simulink model "FLIGHT_Hexacopter_V2"  (R2025a)
settings: Solver=FixedStepDiscrete  StartTime=0.0  StopTime=inf  FixedStep=SampleTime_SAS  RelTol=1e-3  EnableMultiTasking=on
InitFcn:
  | Init_FLIGHT_Hexacopter
values from neighbouring files (symbols this model uses):
  d2r = pi/180    (= 0.0174532925199)    [Init_FLIGHT_Hexacopter.m]
  Kdrr = 0.004    [Init_FLIGHT_Hexacopter_fromNCMS.m]
  Kirr = 0.0    (= 0)    [Init_FLIGHT_Hexacopter_fromNCMS.m]
  Kpp = 3.3894    [Init_FLIGHT_Hexacopter_fromNCMS.m]
  Kpr = 3.3894    [Init_FLIGHT_Hexacopter_fromNCMS.m]
  Kprr = 0.1    [Init_FLIGHT_Hexacopter_fromNCMS.m]
  MAX_CONTROL_ANGLE_PITCH = 30*pi/180    (= 0.523598775598)    [Init_FLIGHT_Hexacopter.m]    (also in Init_FLIGHT_Hexacopter_fromNCMS.m = 0.349065850399)
  MAX_CONTROL_ANGLE_RATE_PITCH = 360*pi/180    (= 6.28318530718)    [Init_FLIGHT_Hexacopter.m]    (also in Init_FLIGHT_Hexacopter_fromNCMS.m)
  MAX_CONTROL_ANGLE_RATE_ROLL = 360*pi/180    (= 6.28318530718)    [Init_FLIGHT_Hexacopter.m]    (also in Init_FLIGHT_Hexacopter_fromNCMS.m)
  MAX_CONTROL_ANGLE_RATE_Y = 120*pi/180    (= 2.09439510239)    [Init_FLIGHT_Hexacopter.m]    (also in Init_FLIGHT_Hexacopter_fromNCMS.m)
  MAX_CONTROL_ANGLE_ROLL = 30*pi/180    (= 0.523598775598)    [Init_FLIGHT_Hexacopter.m]    (also in Init_FLIGHT_Hexacopter_fromNCMS.m = 0.349065850399)
  Nrr = 50    [Init_FLIGHT_Hexacopter_fromNCMS.m]
  PITCH_AUTHORITY = 1    [Init_FLIGHT_Hexacopter.m]
  ROLL_AUTHORITY = 1    [Init_FLIGHT_Hexacopter.m]
  SampleTime = 1/250    (= 0.004)    [Init_FLIGHT_Hexacopter.m]    (also in Init_FLIGHT_Hexacopter_fromNCMS.m = 0.01)
  SampleTime_SAS = 1/1000    (= 0.001)    [Init_FLIGHT_Hexacopter.m]
  YAW_AUTHORITY = 1    [Init_FLIGHT_Hexacopter.m]
undefined symbols (not defined in the file or in its folder): arguments, DiscIntNeverNeededParam, e_dot, event_sequence, fx, g1x, hx, id, integral_e, log_levels, MPC_Z_D, MPC_Z_I, MPC_Z_P, noutputs, omega, omega_dot, output, phi_cmd, phi_cmd_ddot, phi_cmd_dot, r, s, tau_roll, timestamp, w
libraries: px4Utilslib x65, simulink x21, px4uORBlib x12, slpidlib x9, cstblocks x5, simulink_extras x2, sharedtransform x1, px4Sensorslib x1, matrix_library x1, px4Peripheralslib x1
(part 3 of 3)

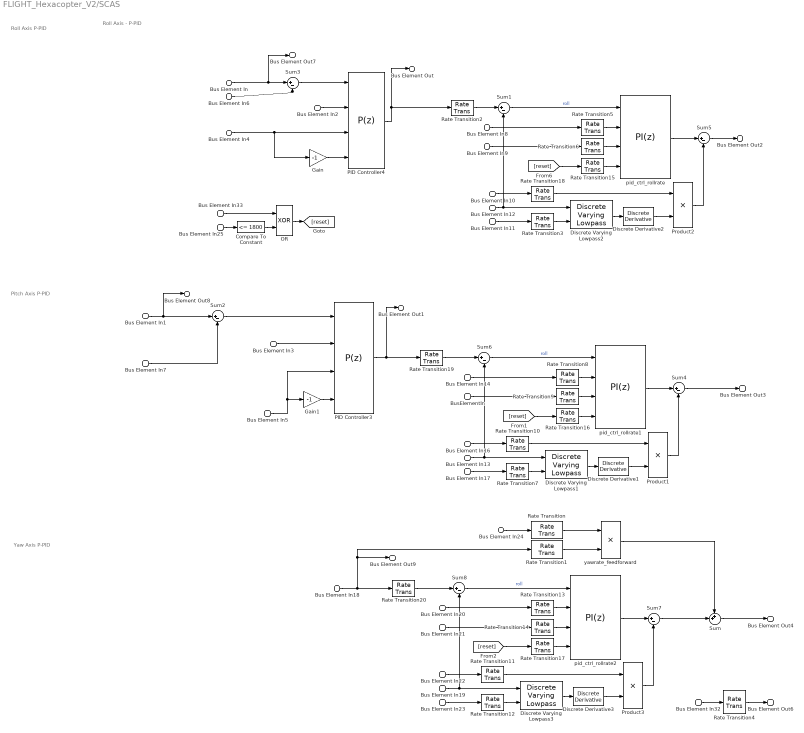
== system FLIGHT_Hexacopter_V2/SCAS ==
  note: Roll Axis P-PID
  note: Roll Axis - P-PID
  note: Pitch Axis P-PID
  note: Yaw Axis P-PID
  Bus Element In : Inport  PortName=OFP  Element=des_roll
  Bus Element In1 : Inport  PortName=OFP  Element=des_pitch
  Bus Element In18 : Inport  PortName=OFP  Element=des_yr
  Bus Element In32 : Inport  PortName=OFP  Element=des_thr
  Bus Element In2 : Inport  Port=2  PortName=PARAMS  Element=MC_ROLL_P
  Bus Element In3 : Inport  Port=2  PortName=PARAMS  Element=MC_PITCH_P
  Bus Element In4 : Inport  Port=2  PortName=PARAMS  Element=MC_ROLLRATE_MAX
  Bus Element In5 : Inport  Port=2  PortName=PARAMS  Element=MC_PITCHRATE_MAX
  Bus Element In8 : Inport  Port=2  PortName=PARAMS  Element=MC_ROLLRATE_P
  Bus Element In9 : Inport  Port=2  PortName=PARAMS  Element=MC_ROLLRATE_I
  Bus Element In10 : Inport  Port=2  PortName=PARAMS  Element=MC_ROLLRATE_D
  Bus Element In11 : Inport  Port=2  PortName=PARAMS  Element=IMU_DGYRO_CUTOFF
  Bus Element In17 : Inport  Port=2  PortName=PARAMS  Element=IMU_DGYRO_CUTOFF
  Bus Element In23 : Inport  Port=2  PortName=PARAMS  Element=IMU_DGYRO_CUTOFF
  Bus Element In14 : Inport  Port=2  PortName=PARAMS  Element=MC_PITCHRATE_P
  Bus Element In16 : Inport  Port=2  PortName=PARAMS  Element=MC_PITCHRATE_D
  Bus Element In20 : Inport  Port=2  PortName=PARAMS  Element=MC_YAWRATE_P
  Bus Element In21 : Inport  Port=2  PortName=PARAMS  Element=MC_YAWRATE_I
  Bus Element In22 : Inport  Port=2  PortName=PARAMS  Element=MC_YAWRATE_D
  Bus Element In24 : Inport  Port=2  PortName=PARAMS  Element=MC_YAWRATE_FF
  BusElementIn : Inport  Port=2  PortName=PARAMS  Element=MC_PITCHRATE_I
  Bus Element In6 : Inport  Port=3  PortName=SENSORS250  Element=Phi
  Bus Element In7 : Inport  Port=3  PortName=SENSORS250  Element=Theta
  Bus Element In33 : Inport  Port=3  PortName=SENSORS250  Element=VehicleStatus_flag_armed
  Bus Element In12 : Inport  Port=4  PortName=SENSORS1000  Element=P
  Bus Element In13 : Inport  Port=4  PortName=SENSORS1000  Element=Q
  Bus Element In19 : Inport  Port=4  PortName=SENSORS1000  Element=R
  Bus Element In25 : Inport  Port=5  PortName=CMD  Element=rc_ctrl_switch
  Compare To Constant : simulink/Logic and Bit Operations/Compare To Constant  relop=<=  const=1800  OutDataTypeStr=boolean
  Discrete Derivative1 : simulink/Discrete/Discrete Derivative  gainval=1.0  ICPrevScaledInput=0.0  OutMin=[]  OutMax=[]  OutDataType=fixdt(1, 16)  OutScaling=2^-10  DoSatur=off
  Discrete Derivative2 : simulink/Discrete/Discrete Derivative  gainval=1.0  ICPrevScaledInput=0.0  OutMin=[]  OutMax=[]  OutDataType=fixdt(1, 16)  OutScaling=2^-10  DoSatur=off
  Discrete Derivative3 : simulink/Discrete/Discrete Derivative  gainval=1.0  ICPrevScaledInput=0.0  OutMin=[]  OutMax=[]  OutDataType=fixdt(1, 16)  OutScaling=2^-10  DoSatur=off
  Discrete Varying Lowpass1 : cstblocks/Linear Parameter Varying/Discrete Varying Lowpass  N=2  w0=0  Ts=SampleTime_SAS
  Discrete Varying Lowpass2 : cstblocks/Linear Parameter Varying/Discrete Varying Lowpass  N=2  w0=0  Ts=SampleTime_SAS
  Discrete Varying Lowpass3 : cstblocks/Linear Parameter Varying/Discrete Varying Lowpass  N=2  w0=0  Ts=SampleTime_SAS
  Gain : Gain  Gain=-1
  Gain1 : Gain  Gain=-1
  OR : Logic  Operator=XOR  AllPortsSameDT=off  OutDataTypeStr=boolean
  PID Controller3 : slpidlib/PID Controller  Controller=P  Form=Parallel  TimeDomain=Discrete-time  UseExternalTs=off  SampleTime=SampleTime  IntegratorMethod=Forward Euler  FilterMethod=Forward Euler  ControllerParametersSource=external  P=Kpp  I=1  UseKiTs=off  D=0  UseExternalDerivativeSource=off  N=100  UseFilter=on  TunerSelectOption=Transfer Function Based (PID Tuner App)  InitialConditionSource=internal  InitialConditionForIntegrator=0  InitialConditionForFilter=0  DifferentiatorICPrevScaledInput=0  ExternalReset=either  TrackingMode=off  Kt=1  LimitOutput=on  SatLimitsSource=external  UpperSaturationLimit=MAX_CONTROL_ANGLE_RATE_PITCH  LowerSaturationLimit=-MAX_CONTROL_ANGLE_RATE_PITCH  LinearizeAsGain=on  AntiWindupMode=clamping  Kb=1  LimitIntegrator=on  UpperIntegratorSaturationLimit=220*d2r*0.3  LowerIntegratorSaturationLimit=-220*d2r*0.3  POutMin=[]  POutMax=[]  IOutMin=[]  IOutMax=[]  DOutMin=[]  DOutMax=[]  NOutMin=[]  NOutMax=[]  SumOutMin=[]  SumOutMax=[]  SaturationOutMin=[]  SaturationOutMax=[]  PParamMin=[]  PParamMax=[]  IParamMin=[]  IParamMax=[]  DParamMin=[]  DParamMax=[]  NParamMin=[]  NParamMax=[]  KbParamMin=[]  KbParamMax=[]  KtParamMin=[]  KtParamMax=[]  KbOutMin=[]  KbOutMax=[]  KtOutMin=[]  KtOutMax=[]  IntegratorOutMin=[]  IntegratorOutMax=[]  FilterOutMin=[]  FilterOutMax=[]  SumI1OutMin=[]  SumI1OutMax=[]  SumI2OutMin=[]  SumI2OutMax=[]  SumI3OutMin=[]  SumI3OutMax=[]  SumI4OutMin=[]  SumI4OutMax=[]  SumDOutMin=[]  SumDOutMax=[]  DifferentiatorOutMin=[]  DifferentiatorOutMax=[]  FilterDiffOutCoefMin=[]  FilterDiffOutCoefMax=[]  ReciprocalOutMin=[]  ReciprocalOutMax=[]  SumDenOutMin=[]  SumDenOutMax=[]  SumNumOutMin=[]  SumNumOutMax=[]  DivideOutMin=[]  DivideOutMax=[]  UdiffTsProdOutMin=[]  UdiffTsProdOutMax=[]  NTsProdOutMin=[]  NTsProdOutMax=[]  UintegralTsProdOutMin=[]  UintegralTsProdOutMax=[]  UngainTsProdOutMin=[]  UngainTsProdOutMax=[]  ClampingZeroOutDataTypeStr=Inherit: Inherit via back propagation  ClampingZeroOutMin=[]  ClampingZeroOutMax=[]  FilterDenConstantOutDataTypeStr=Inherit: Inherit via back propagation  FilterDenConstantOutMin=[]  FilterDenConstantOutMax=[]  PCopyOutDataTypeStr=Inherit: Inherit via back propagation  PCopyOutMin=[]  PCopyOutMax=[]  NCopyOutDataTypeStr=Inherit: Inherit via back propagation  NCopyOutMin=[]  NCopyOutMax=[]  IntegratorContinuousStateAttributes=''  IntegratorStateMustResolveToSignalObject=off  IntegratorRTWStateStorageClass=Auto  FilterContinuousStateAttributes=''  FilterStateMustResolveToSignalObject=off  FilterRTWStateStorageClass=Auto  ParallelPVariant=ExternalParameters  IdealPVariant=Disabled  IVariant=Disabled  DVariant=Disabled  IntegratorVariant=Disabled  SatVariant=External  AWVariant=Disabled  PCopyVariant=Disabled  TRVariant=Disabled  FdbkBlocksVariant=Forward  IdealPFdbkVariant=Disabled  SatFdbkVariant=Disabled  DerivativeFilterVariant=Disabled  NVariant=Disabled  NCopyVariant=Disabled_SignalSpec  FilterICVariant=Disabled  IntegratorICVariant=Disabled  ExternalResetVariant=Disabled  TRSumVariant=Passthrough  SumFdbkVariant=Disabled  SumVariant=Passthrough_P  TsampFilterVariant=InternalTs  TsampNgainVariant=Passthrough  TsampIntegralVariant=Disabled_SignalSpec  ExternalSaturationOutDataTypeStr=Inherit: Same as second input  DerivativeSourceVariant=Disabled  PreIntVariant=InternalPreInt
  PID Controller4 : slpidlib/PID Controller  Controller=P  Form=Parallel  TimeDomain=Discrete-time  UseExternalTs=off  SampleTime=SampleTime  IntegratorMethod=Forward Euler  FilterMethod=Forward Euler  ControllerParametersSource=external  P=Kpr  I=1  UseKiTs=off  D=0  UseExternalDerivativeSource=off  N=100  UseFilter=on  TunerSelectOption=Transfer Function Based (PID Tuner App)  InitialConditionSource=internal  InitialConditionForIntegrator=0  InitialConditionForFilter=0  DifferentiatorICPrevScaledInput=0  ExternalReset=either  TrackingMode=off  Kt=1  LimitOutput=on  SatLimitsSource=external  UpperSaturationLimit=MAX_CONTROL_ANGLE_RATE_ROLL  LowerSaturationLimit=-MAX_CONTROL_ANGLE_RATE_ROLL  LinearizeAsGain=on  AntiWindupMode=clamping  Kb=1  LimitIntegrator=on  UpperIntegratorSaturationLimit=220*d2r*0.3  LowerIntegratorSaturationLimit=-220*d2r*0.3  POutMin=[]  POutMax=[]  IOutMin=[]  IOutMax=[]  DOutMin=[]  DOutMax=[]  NOutMin=[]  NOutMax=[]  SumOutMin=[]  SumOutMax=[]  SaturationOutMin=[]  SaturationOutMax=[]  PParamMin=[]  PParamMax=[]  IParamMin=[]  IParamMax=[]  DParamMin=[]  DParamMax=[]  NParamMin=[]  NParamMax=[]  KbParamMin=[]  KbParamMax=[]  KtParamMin=[]  KtParamMax=[]  KbOutMin=[]  KbOutMax=[]  KtOutMin=[]  KtOutMax=[]  IntegratorOutMin=[]  IntegratorOutMax=[]  FilterOutMin=[]  FilterOutMax=[]  SumI1OutMin=[]  SumI1OutMax=[]  SumI2OutMin=[]  SumI2OutMax=[]  SumI3OutMin=[]  SumI3OutMax=[]  SumI4OutMin=[]  SumI4OutMax=[]  SumDOutMin=[]  SumDOutMax=[]  DifferentiatorOutMin=[]  DifferentiatorOutMax=[]  FilterDiffOutCoefMin=[]  FilterDiffOutCoefMax=[]  ReciprocalOutMin=[]  ReciprocalOutMax=[]  SumDenOutMin=[]  SumDenOutMax=[]  SumNumOutMin=[]  SumNumOutMax=[]  DivideOutMin=[]  DivideOutMax=[]  UdiffTsProdOutMin=[]  UdiffTsProdOutMax=[]  NTsProdOutMin=[]  NTsProdOutMax=[]  UintegralTsProdOutMin=[]  UintegralTsProdOutMax=[]  UngainTsProdOutMin=[]  UngainTsProdOutMax=[]  ClampingZeroOutDataTypeStr=Inherit: Inherit via back propagation  ClampingZeroOutMin=[]  ClampingZeroOutMax=[]  FilterDenConstantOutDataTypeStr=Inherit: Inherit via back propagation  FilterDenConstantOutMin=[]  FilterDenConstantOutMax=[]  PCopyOutDataTypeStr=Inherit: Inherit via back propagation  PCopyOutMin=[]  PCopyOutMax=[]  NCopyOutDataTypeStr=Inherit: Inherit via back propagation  NCopyOutMin=[]  NCopyOutMax=[]  IntegratorContinuousStateAttributes=''  IntegratorStateMustResolveToSignalObject=off  IntegratorRTWStateStorageClass=Auto  FilterContinuousStateAttributes=''  FilterStateMustResolveToSignalObject=off  FilterRTWStateStorageClass=Auto  ParallelPVariant=ExternalParameters  IdealPVariant=Disabled  IVariant=Disabled  DVariant=Disabled  IntegratorVariant=Disabled  SatVariant=External  AWVariant=Disabled  PCopyVariant=Disabled  TRVariant=Disabled  FdbkBlocksVariant=Forward  IdealPFdbkVariant=Disabled  SatFdbkVariant=Disabled  DerivativeFilterVariant=Disabled  NVariant=Disabled  NCopyVariant=Disabled_SignalSpec  FilterICVariant=Disabled  IntegratorICVariant=Disabled  ExternalResetVariant=Disabled  TRSumVariant=Passthrough  SumFdbkVariant=Disabled  SumVariant=Passthrough_P  TsampFilterVariant=InternalTs  TsampNgainVariant=Passthrough  TsampIntegralVariant=Disabled_SignalSpec  ExternalSaturationOutDataTypeStr=Inherit: Same as second input  DerivativeSourceVariant=Disabled  PreIntVariant=InternalPreInt
  Product1 : Product
  Product2 : Product
  Product3 : Product
  Rate Transition{,1..20} (21 alike) : RateTransition  OutPortSampleTime=SampleTime_SAS
  Sum : Sum  Inputs=++|
  Sum{1..8} (8 alike) : Sum  Inputs=|+-
  pid_ctrl_rollrate : slpidlib/PID Controller  Controller=PI  Form=Parallel  TimeDomain=Discrete-time  UseExternalTs=off  SampleTime=SampleTime_SAS  IntegratorMethod=Forward Euler  FilterMethod=Forward Euler  ControllerParametersSource=external  P=Kprr  I=Kirr  UseKiTs=off  D=Kdrr  UseExternalDerivativeSource=off  N=Nrr  UseFilter=on  TunerSelectOption=Transfer Function Based (PID Tuner App)  InitialConditionSource=internal  InitialConditionForIntegrator=0  InitialConditionForFilter=0  DifferentiatorICPrevScaledInput=0  ExternalReset=either  TrackingMode=off  Kt=1  LimitOutput=on  SatLimitsSource=internal  UpperSaturationLimit=abs(ROLL_AUTHORITY)  LowerSaturationLimit=-abs(ROLL_AUTHORITY)  LinearizeAsGain=on  AntiWindupMode=clamping  Kb=1  LimitIntegrator=on  UpperIntegratorSaturationLimit=abs(ROLL_AUTHORITY)*0.3  LowerIntegratorSaturationLimit=-abs(ROLL_AUTHORITY)*0.3  SaturateOnIntegerOverflow=on  POutMin=[]  POutMax=[]  IOutMin=[]  IOutMax=[]  DOutMin=[]  DOutMax=[]  NOutMin=[]  NOutMax=[]  SumOutMin=[]  SumOutMax=[]  SaturationOutDataTypeStr=single  SaturationOutMin=[]  SaturationOutMax=[]  PParamMin=[]  PParamMax=[]  IParamMin=[]  IParamMax=[]  DParamMin=[]  DParamMax=[]  NParamMin=[]  NParamMax=[]  KbParamMin=[]  KbParamMax=[]  KtParamMin=[]  KtParamMax=[]  KbOutMin=[]  KbOutMax=[]  KtOutMin=[]  KtOutMax=[]  IntegratorOutMin=[]  IntegratorOutMax=[]  FilterOutMin=[]  FilterOutMax=[]  SumI1OutMin=[]  SumI1OutMax=[]  SumI2OutMin=[]  SumI2OutMax=[]  SumI3OutMin=[]  SumI3OutMax=[]  SumI4OutMin=[]  SumI4OutMax=[]  SumDOutMin=[]  SumDOutMax=[]  DifferentiatorOutMin=[]  DifferentiatorOutMax=[]  FilterDiffOutCoefMin=[]  FilterDiffOutCoefMax=[]  ReciprocalOutMin=[]  ReciprocalOutMax=[]  SumDenOutMin=[]  SumDenOutMax=[]  SumNumOutMin=[]  SumNumOutMax=[]  DivideOutMin=[]  DivideOutMax=[]  UdiffTsProdOutMin=[]  UdiffTsProdOutMax=[]  NTsProdOutMin=[]  NTsProdOutMax=[]  UintegralTsProdOutMin=[]  UintegralTsProdOutMax=[]  UngainTsProdOutMin=[]  UngainTsProdOutMax=[]  ClampingZeroOutDataTypeStr=Inherit: Inherit via back propagation  ClampingZeroOutMin=[]  ClampingZeroOutMax=[]  FilterDenConstantOutDataTypeStr=Inherit: Inherit via back propagation  FilterDenConstantOutMin=[]  FilterDenConstantOutMax=[]  PCopyOutDataTypeStr=Inherit: Inherit via back propagation  PCopyOutMin=[]  PCopyOutMax=[]  NCopyOutDataTypeStr=Inherit: Inherit via back propagation  NCopyOutMin=[]  NCopyOutMax=[]  IntegratorContinuousStateAttributes=''  IntegratorStateMustResolveToSignalObject=off  IntegratorRTWStateStorageClass=Auto  FilterContinuousStateAttributes=''  FilterStateMustResolveToSignalObject=off  FilterRTWStateStorageClass=Auto  ParallelPVariant=ExternalParameters  IdealPVariant=Disabled  IVariant=ExternalParameters  DVariant=Disabled  IntegratorVariant=Discrete  SatVariant=Enabled  AWVariant=DiscClampingParallel  PCopyVariant=Disabled  TRVariant=Disabled  FdbkBlocksVariant=Forward  IdealPFdbkVariant=Disabled  SatFdbkVariant=Disabled  DerivativeFilterVariant=Disabled  NVariant=Disabled  NCopyVariant=Disabled_SignalSpec  FilterICVariant=Disabled  IntegratorICVariant=InternalICs  ExternalResetVariant=ExternalReset  TRSumVariant=Passthrough  SumFdbkVariant=Disabled  SumVariant=Sum_PI  TsampFilterVariant=InternalTs  TsampNgainVariant=Passthrough  TsampIntegralVariant=Disabled_SignalSpec  ExternalSaturationOutDataTypeStr=single  DerivativeSourceVariant=Disabled  PreIntVariant=InternalPreInt
  pid_ctrl_rollrate1 : slpidlib/PID Controller  Controller=PI  Form=Parallel  TimeDomain=Discrete-time  UseExternalTs=off  SampleTime=SampleTime_SAS  IntegratorMethod=Forward Euler  FilterMethod=Forward Euler  ControllerParametersSource=external  P=Kprr  I=Kirr  UseKiTs=off  D=Kdrr  UseExternalDerivativeSource=off  N=Nrr  UseFilter=on  TunerSelectOption=Transfer Function Based (PID Tuner App)  InitialConditionSource=internal  InitialConditionForIntegrator=0  InitialConditionForFilter=0  DifferentiatorICPrevScaledInput=0  ExternalReset=either  TrackingMode=off  Kt=1  LimitOutput=on  SatLimitsSource=internal  UpperSaturationLimit=abs(PITCH_AUTHORITY)  LowerSaturationLimit=-abs(PITCH_AUTHORITY)  LinearizeAsGain=on  AntiWindupMode=clamping  Kb=1  LimitIntegrator=on  UpperIntegratorSaturationLimit=abs(PITCH_AUTHORITY)*0.3  LowerIntegratorSaturationLimit=-abs(PITCH_AUTHORITY)*0.3  SaturateOnIntegerOverflow=on  POutMin=[]  POutMax=[]  IOutMin=[]  IOutMax=[]  DOutMin=[]  DOutMax=[]  NOutMin=[]  NOutMax=[]  SumOutMin=[]  SumOutMax=[]  SaturationOutDataTypeStr=single  SaturationOutMin=[]  SaturationOutMax=[]  PParamMin=[]  PParamMax=[]  IParamMin=[]  IParamMax=[]  DParamMin=[]  DParamMax=[]  NParamMin=[]  NParamMax=[]  KbParamMin=[]  KbParamMax=[]  KtParamMin=[]  KtParamMax=[]  KbOutMin=[]  KbOutMax=[]  KtOutMin=[]  KtOutMax=[]  IntegratorOutMin=[]  IntegratorOutMax=[]  FilterOutMin=[]  FilterOutMax=[]  SumI1OutMin=[]  SumI1OutMax=[]  SumI2OutMin=[]  SumI2OutMax=[]  SumI3OutMin=[]  SumI3OutMax=[]  SumI4OutMin=[]  SumI4OutMax=[]  SumDOutMin=[]  SumDOutMax=[]  DifferentiatorOutMin=[]  DifferentiatorOutMax=[]  FilterDiffOutCoefMin=[]  FilterDiffOutCoefMax=[]  ReciprocalOutMin=[]  ReciprocalOutMax=[]  SumDenOutMin=[]  SumDenOutMax=[]  SumNumOutMin=[]  SumNumOutMax=[]  DivideOutMin=[]  DivideOutMax=[]  UdiffTsProdOutMin=[]  UdiffTsProdOutMax=[]  NTsProdOutMin=[]  NTsProdOutMax=[]  UintegralTsProdOutMin=[]  UintegralTsProdOutMax=[]  UngainTsProdOutMin=[]  UngainTsProdOutMax=[]  ClampingZeroOutDataTypeStr=Inherit: Inherit via back propagation  ClampingZeroOutMin=[]  ClampingZeroOutMax=[]  FilterDenConstantOutDataTypeStr=Inherit: Inherit via back propagation  FilterDenConstantOutMin=[]  FilterDenConstantOutMax=[]  PCopyOutDataTypeStr=Inherit: Inherit via back propagation  PCopyOutMin=[]  PCopyOutMax=[]  NCopyOutDataTypeStr=Inherit: Inherit via back propagation  NCopyOutMin=[]  NCopyOutMax=[]  IntegratorContinuousStateAttributes=''  IntegratorStateMustResolveToSignalObject=off  IntegratorRTWStateStorageClass=Auto  FilterContinuousStateAttributes=''  FilterStateMustResolveToSignalObject=off  FilterRTWStateStorageClass=Auto  ParallelPVariant=ExternalParameters  IdealPVariant=Disabled  IVariant=ExternalParameters  DVariant=Disabled  IntegratorVariant=Discrete  SatVariant=Enabled  AWVariant=DiscClampingParallel  PCopyVariant=Disabled  TRVariant=Disabled  FdbkBlocksVariant=Forward  IdealPFdbkVariant=Disabled  SatFdbkVariant=Disabled  DerivativeFilterVariant=Disabled  NVariant=Disabled  NCopyVariant=Disabled_SignalSpec  FilterICVariant=Disabled  IntegratorICVariant=InternalICs  ExternalResetVariant=ExternalReset  TRSumVariant=Passthrough  SumFdbkVariant=Disabled  SumVariant=Sum_PI  TsampFilterVariant=InternalTs  TsampNgainVariant=Passthrough  TsampIntegralVariant=Disabled_SignalSpec  ExternalSaturationOutDataTypeStr=single  DerivativeSourceVariant=Disabled  PreIntVariant=InternalPreInt
  pid_ctrl_rollrate2 : slpidlib/PID Controller  Controller=PI  Form=Parallel  TimeDomain=Discrete-time  UseExternalTs=off  SampleTime=SampleTime_SAS  IntegratorMethod=Forward Euler  FilterMethod=Forward Euler  ControllerParametersSource=external  P=Kprr  I=Kirr  UseKiTs=off  D=Kdrr  UseExternalDerivativeSource=off  N=Nrr  UseFilter=on  TunerSelectOption=Transfer Function Based (PID Tuner App)  InitialConditionSource=internal  InitialConditionForIntegrator=0  InitialConditionForFilter=0  DifferentiatorICPrevScaledInput=0  ExternalReset=either  TrackingMode=off  Kt=1  LimitOutput=on  SatLimitsSource=internal  UpperSaturationLimit=abs(YAW_AUTHORITY)  LowerSaturationLimit=-abs(YAW_AUTHORITY)  LinearizeAsGain=on  AntiWindupMode=clamping  Kb=1  LimitIntegrator=on  UpperIntegratorSaturationLimit=abs(YAW_AUTHORITY)*0.3  LowerIntegratorSaturationLimit=-abs(YAW_AUTHORITY)*0.3  SaturateOnIntegerOverflow=on  POutMin=[]  POutMax=[]  IOutMin=[]  IOutMax=[]  DOutMin=[]  DOutMax=[]  NOutMin=[]  NOutMax=[]  SumOutMin=[]  SumOutMax=[]  SaturationOutDataTypeStr=single  SaturationOutMin=[]  SaturationOutMax=[]  PParamMin=[]  PParamMax=[]  IParamMin=[]  IParamMax=[]  DParamMin=[]  DParamMax=[]  NParamMin=[]  NParamMax=[]  KbParamMin=[]  KbParamMax=[]  KtParamMin=[]  KtParamMax=[]  KbOutMin=[]  KbOutMax=[]  KtOutMin=[]  KtOutMax=[]  IntegratorOutMin=[]  IntegratorOutMax=[]  FilterOutMin=[]  FilterOutMax=[]  SumI1OutMin=[]  SumI1OutMax=[]  SumI2OutMin=[]  SumI2OutMax=[]  SumI3OutMin=[]  SumI3OutMax=[]  SumI4OutMin=[]  SumI4OutMax=[]  SumDOutMin=[]  SumDOutMax=[]  DifferentiatorOutMin=[]  DifferentiatorOutMax=[]  FilterDiffOutCoefMin=[]  FilterDiffOutCoefMax=[]  ReciprocalOutMin=[]  ReciprocalOutMax=[]  SumDenOutMin=[]  SumDenOutMax=[]  SumNumOutMin=[]  SumNumOutMax=[]  DivideOutMin=[]  DivideOutMax=[]  UdiffTsProdOutMin=[]  UdiffTsProdOutMax=[]  NTsProdOutMin=[]  NTsProdOutMax=[]  UintegralTsProdOutMin=[]  UintegralTsProdOutMax=[]  UngainTsProdOutMin=[]  UngainTsProdOutMax=[]  ClampingZeroOutDataTypeStr=Inherit: Inherit via back propagation  ClampingZeroOutMin=[]  ClampingZeroOutMax=[]  FilterDenConstantOutDataTypeStr=Inherit: Inherit via back propagation  FilterDenConstantOutMin=[]  FilterDenConstantOutMax=[]  PCopyOutDataTypeStr=Inherit: Inherit via back propagation  PCopyOutMin=[]  PCopyOutMax=[]  NCopyOutDataTypeStr=Inherit: Inherit via back propagation  NCopyOutMin=[]  NCopyOutMax=[]  IntegratorContinuousStateAttributes=''  IntegratorStateMustResolveToSignalObject=off  IntegratorRTWStateStorageClass=Auto  FilterContinuousStateAttributes=''  FilterStateMustResolveToSignalObject=off  FilterRTWStateStorageClass=Auto  ParallelPVariant=ExternalParameters  IdealPVariant=Disabled  IVariant=ExternalParameters  DVariant=Disabled  IntegratorVariant=Discrete  SatVariant=Enabled  AWVariant=DiscClampingParallel  PCopyVariant=Disabled  TRVariant=Disabled  FdbkBlocksVariant=Forward  IdealPFdbkVariant=Disabled  SatFdbkVariant=Disabled  DerivativeFilterVariant=Disabled  NVariant=Disabled  NCopyVariant=Disabled_SignalSpec  FilterICVariant=Disabled  IntegratorICVariant=InternalICs  ExternalResetVariant=ExternalReset  TRSumVariant=Passthrough  SumFdbkVariant=Disabled  SumVariant=Sum_PI  TsampFilterVariant=InternalTs  TsampNgainVariant=Passthrough  TsampIntegralVariant=Disabled_SignalSpec  ExternalSaturationOutDataTypeStr=single  DerivativeSourceVariant=Disabled  PreIntVariant=InternalPreInt
  yawrate_feedforward : Product
  Bus Element Out : Outport  PortName=SCAS  Element=des_rollrate
  Bus Element Out1 : Outport  PortName=SCAS  Element=des_pitchrate
  Bus Element Out2 : Outport  PortName=SCAS  Element=tau_roll
  Bus Element Out3 : Outport  PortName=SCAS  Element=tau_pitch
  Bus Element Out4 : Outport  PortName=SCAS  Element=tau_yaw
  Bus Element Out6 : Outport  PortName=SCAS  Element=tau_throttle
  Bus Element Out7 : Outport  PortName=SCAS  Element=des_roll
  Bus Element Out8 : Outport  PortName=SCAS  Element=des_pitch
  Bus Element Out9 : Outport  PortName=SCAS  Element=des_yr
  wires:
  Bus Element In4/1 -> Gain/1, PID Controller4/3
  Gain/1 -> PID Controller4/4
  Bus Element In3/1 -> PID Controller3/2
  Bus Element In/1 -> Bus Element Out7/1, Sum3/1
  Sum2/1 -> PID Controller3/1
  Gain1/1 -> PID Controller3/4
  Bus Element In2/1 -> PID Controller4/2
  Sum3/1 -> PID Controller4/1
  Bus Element In5/1 -> PID Controller3/3, Gain1/1
  Bus Element In1/1 -> Bus Element Out8/1, Sum2/1
  Bus Element In6/1 -> Sum3/2
  Bus Element In7/1 -> Sum2/2
  PID Controller3/1 -> Rate Transition19/1, Bus Element Out1/1
  Bus Element In18/1 -> Rate Transition20/1, Rate Transition1/1, Bus Element Out9/1
  yawrate_feedforward/1 -> Sum/1
  Bus Element In24/1 -> Rate Transition/1
  Sum7/1 -> Sum/2
  Sum/1 -> Bus Element Out4/1
  Sum4/1 -> Bus Element Out3/1
  Sum5/1 -> Bus Element Out2/1
  Rate Transition/1 -> yawrate_feedforward/1
  Rate Transition1/1 -> yawrate_feedforward/2
  Bus Element In32/1 -> Rate Transition4/1
  Rate Transition4/1 -> Bus Element Out6/1
  Bus Element In33/1 -> OR/1
  Bus Element In25/1 -> Compare To Constant/1
  Compare To Constant/1 -> OR/2
  OR/1 -> [reset]
  Rate Transition5/1 -> pid_ctrl_rollrate/2
  Bus Element In12/1 -> Discrete Varying Lowpass2/1, Sum1/2
  PID Controller4/1 -> Bus Element Out/1, Rate Transition2/1
  [reset] -> Rate Transition15/1
  Discrete Varying Lowpass2/1 -> Discrete Derivative2/1
  pid_ctrl_rollrate/1 -> Sum5/1
  Discrete Derivative2/1 -> Product2/2
  Product2/1 -> Sum5/2
  Sum1/1 -> pid_ctrl_rollrate/1  "roll"
  Bus Element In11/1 -> Rate Transition3/1
  Rate Transition2/1 -> Sum1/1
  Bus Element In10/1 -> Rate Transition18/1
  Rate Transition6/1 -> pid_ctrl_rollrate/3
  Rate Transition3/1 -> Discrete Varying Lowpass2/2
  Bus Element In8/1 -> Rate Transition5/1
  Bus Element In9/1 -> Rate Transition6/1
  Rate Transition8/1 -> pid_ctrl_rollrate1/2
  Discrete Derivative1/1 -> Product1/2
  Rate Transition9/1 -> pid_ctrl_rollrate1/3
  [reset] -> Rate Transition16/1
  Bus Element In14/1 -> Rate Transition8/1
  Bus Element In17/1 -> Rate Transition7/1
  pid_ctrl_rollrate1/1 -> Sum4/1
  Rate Transition7/1 -> Discrete Varying Lowpass1/2
  Discrete Varying Lowpass1/1 -> Discrete Derivative1/1
  BusElementIn/1 -> Rate Transition9/1
  Product1/1 -> Sum4/2
  Sum6/1 -> pid_ctrl_rollrate1/1  "roll"
  Bus Element In13/1 -> Discrete Varying Lowpass1/1, Sum6/2
  Bus Element In16/1 -> Rate Transition10/1
  Rate Transition10/1 -> Product1/1
  Rate Transition13/1 -> pid_ctrl_rollrate2/2
  Bus Element In19/1 -> Discrete Varying Lowpass3/1, Sum8/2
  Product3/1 -> Sum7/2
  Rate Transition14/1 -> pid_ctrl_rollrate2/3
  Rate Transition12/1 -> Discrete Varying Lowpass3/2
  Rate Transition11/1 -> Product3/1
  pid_ctrl_rollrate2/1 -> Sum7/1
  Bus Element In22/1 -> Rate Transition11/1
  Discrete Varying Lowpass3/1 -> Discrete Derivative3/1
  Bus Element In21/1 -> Rate Transition14/1
  [reset] -> Rate Transition17/1
  Sum8/1 -> pid_ctrl_rollrate2/1  "roll"
  Discrete Derivative3/1 -> Product3/2
  Bus Element In20/1 -> Rate Transition13/1
  Bus Element In23/1 -> Rate Transition12/1
  Rate Transition15/1 -> pid_ctrl_rollrate/4
  Rate Transition16/1 -> pid_ctrl_rollrate1/4
  Rate Transition17/1 -> pid_ctrl_rollrate2/4
  Rate Transition18/1 -> Product2/1
  Rate Transition19/1 -> Sum6/1
  Rate Transition20/1 -> Sum8/1

== system FLIGHT_Hexacopter_V2/Subsystem ==
  BusElementIn1 : Inport  PortName=CA  Element=thr_m1
  BusElementIn2 : Inport  PortName=CA  Element=thr_m2
  BusElementIn3 : Inport  PortName=CA  Element=thr_m3
  BusElementIn4 : Inport  PortName=CA  Element=thr_m4
  BusElementIn5 : Inport  PortName=CA  Element=thr_m5
  BusElementIn8 : Inport  PortName=CA  Element=thr_m6
  BusElementIn6 : Inport  Port=2  PortName=SENSOR250  Element=VehicleStatus_armed
  BusElementIn : Inport  Port=2  PortName=SENSOR250  Element=VehicleStatus_emergency_kill
  Constant : Constant  Value=false  OutDataTypeStr=boolean  SampleTime=SampleTime_SAS
  NOT : Logic  Operator=NOT  IconShape=distinctive  AllPortsSameDT=off  OutDataTypeStr=boolean
  PX4 Actuator Write : px4Peripheralslib/PX4 Actuator Write  Motor1Enable=on  Motor2Enable=on  Motor3Enable=on  Motor4Enable=on  Motor5Enable=on  Motor6Enable=on  Motor7Enable=off  Motor8Enable=off  Motor9Enable=off  Motor10Enable=off  Motor11Enable=off  Motor12Enable=off  IsMotorArray=off  Servo1Enable=off  Servo2Enable=off  Servo3Enable=off  Servo4Enable=off  Servo5Enable=off  Servo6Enable=off  Servo7Enable=off  Servo8Enable=off  IsServoArray=off
  Switch : Switch  Criteria=u2 ~= 0  SaturateOnIntegerOverflow=off  InputSameDT=off
  wires:
  BusElementIn8/1 -> PX4 Actuator Write/7
  BusElementIn5/1 -> PX4 Actuator Write/6
  BusElementIn4/1 -> PX4 Actuator Write/5
  BusElementIn3/1 -> PX4 Actuator Write/4
  BusElementIn2/1 -> PX4 Actuator Write/3
  BusElementIn1/1 -> PX4 Actuator Write/2
  BusElementIn/1 -> NOT/1
  BusElementIn6/1 -> Switch/1
  Constant/1 -> Switch/3
  Switch/1 -> PX4 Actuator Write/1
  NOT/1 -> Switch/2

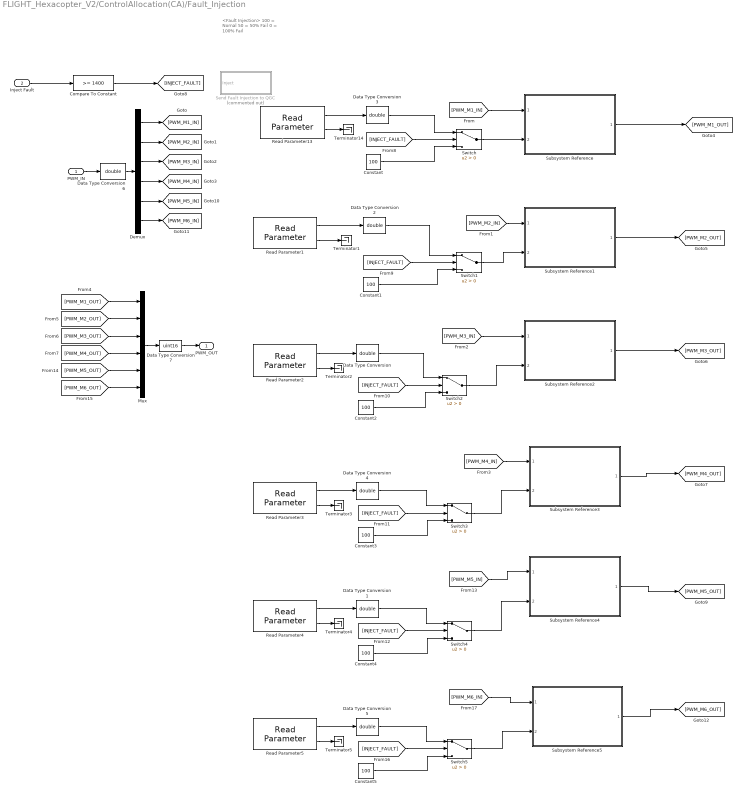
== system FLIGHT_Hexacopter_V2/ControlAllocation(CA)/Fault_Injection ==
  note: <Fault Injection>
      | 100 = Nornal
      | 50 = 50% Fail
      | 0 = 100% Fail
  PWM_IN : Inport
  Inject Fault : Inport  Port=2
  Compare To Constant : simulink/Logic and Bit Operations/Compare To Constant  relop=>=  const=1400  OutDataTypeStr=boolean
  Constant{,1..5} (6 alike) : Constant  Value=100
  Data Type Conversion{,1..6} (7 alike) : DataTypeConversion  OutDataTypeStr=double  SaturateOnIntegerOverflow=off  RndMeth=Floor
  Data Type Conversion7 : DataTypeConversion  OutDataTypeStr=uint16  SaturateOnIntegerOverflow=off  RndMeth=Floor
  Demux : Demux  Outputs=6
  Mux : Mux  Inputs=6
  Read Parameter1 : px4Utilslib/Read Parameter  ParameterName=FDD_M2_STATUS  DataType=INT32  SampleTime=SampleTime_SAS
  Read Parameter13 : px4Utilslib/Read Parameter  ParameterName=FDD_M1_STATUS  DataType=INT32  SampleTime=SampleTime_SAS
  Read Parameter2 : px4Utilslib/Read Parameter  ParameterName=FDD_M3_STATUS  DataType=INT32  SampleTime=SampleTime_SAS
  Read Parameter3 : px4Utilslib/Read Parameter  ParameterName=FDD_M4_STATUS  DataType=INT32  SampleTime=SampleTime_SAS
  Read Parameter4 : px4Utilslib/Read Parameter  ParameterName=FDD_M5_STATUS  DataType=INT32  SampleTime=SampleTime_SAS
  Read Parameter5 : px4Utilslib/Read Parameter  ParameterName=FDD_M6_STATUS  DataType=INT32  SampleTime=SampleTime_SAS
  Send Fault Injection to QGC : Subsystem  Commented=on  TreatAsAtomicUnit=on
  Subsystem Reference{,1..5} (6 alike) : Subsystem  ReferencedSubsystem=calculate_fault_injected_pwm
  Switch{,1..5} (6 alike) : Switch  Criteria=u2 > Threshold  SaturateOnIntegerOverflow=off  InputSameDT=off
  Terminator{1..5,14} (6 alike) : Terminator
  PWM_OUT : Outport
  wires:
  Read Parameter13/2 -> Terminator14/1
  Read Parameter1/2 -> Terminator1/1
  Read Parameter2/2 -> Terminator2/1
  Read Parameter2/1 -> Data Type Conversion/1
  Read Parameter3/2 -> Terminator3/1
  Read Parameter3/1 -> Data Type Conversion4/1
  Read Parameter13/1 -> Data Type Conversion3/1
  Read Parameter1/1 -> Data Type Conversion2/1
  Demux/1 -> [PWM_M1_IN]
  Demux/2 -> [PWM_M2_IN]
  Demux/3 -> [PWM_M3_IN]
  Demux/4 -> [PWM_M4_IN]
  Mux/1 -> Data Type Conversion7/1
  [PWM_M1_OUT] -> Mux/1
  [PWM_M2_OUT] -> Mux/2
  [PWM_M3_OUT] -> Mux/3
  [PWM_M4_OUT] -> Mux/4
  Inject Fault/1 -> Compare To Constant/1
  Compare To Constant/1 -> [INJECT_FAULT]
  Data Type Conversion3/1 -> Switch/1
  [INJECT_FAULT] -> Switch/2
  Constant/1 -> Switch/3
  Constant1/1 -> Switch1/3
  [INJECT_FAULT] -> Switch1/2
  Constant2/1 -> Switch2/3
  [INJECT_FAULT] -> Switch2/2
  Data Type Conversion/1 -> Switch2/1
  Constant3/1 -> Switch3/3
  [INJECT_FAULT] -> Switch3/2
  Data Type Conversion4/1 -> Switch3/1
  Read Parameter4/1 -> Data Type Conversion1/1
  Data Type Conversion1/1 -> Switch4/1
  Constant4/1 -> Switch4/3
  Read Parameter4/2 -> Terminator4/1
  [INJECT_FAULT] -> Switch4/2
  Demux/5 -> [PWM_M5_IN]
  Demux/6 -> [PWM_M6_IN]
  [PWM_M5_OUT] -> Mux/5
  [PWM_M6_OUT] -> Mux/6
  Data Type Conversion5/1 -> Switch5/1
  Read Parameter5/2 -> Terminator5/1
  [INJECT_FAULT] -> Switch5/2
  Read Parameter5/1 -> Data Type Conversion5/1
  Constant5/1 -> Switch5/3
  Data Type Conversion2/1 -> Switch1/1
  [PWM_M1_IN] -> Subsystem Reference/1
  Switch/1 -> Subsystem Reference/2
  [PWM_M2_IN] -> Subsystem Reference1/1
  Switch1/1 -> Subsystem Reference1/2
  [PWM_M3_IN] -> Subsystem Reference2/1
  Switch2/1 -> Subsystem Reference2/2
  Switch3/1 -> Subsystem Reference3/2
  [PWM_M4_IN] -> Subsystem Reference3/1
  [PWM_M5_IN] -> Subsystem Reference4/1
  Switch4/1 -> Subsystem Reference4/2
  [PWM_M6_IN] -> Subsystem Reference5/1
  Switch5/1 -> Subsystem Reference5/2
  Subsystem Reference/1 -> [PWM_M1_OUT]
  Subsystem Reference1/1 -> [PWM_M2_OUT]
  Subsystem Reference2/1 -> [PWM_M3_OUT]
  Subsystem Reference3/1 -> [PWM_M4_OUT]
  Subsystem Reference4/1 -> [PWM_M5_OUT]
  Subsystem Reference5/1 -> [PWM_M6_OUT]
  Data Type Conversion6/1 -> Demux/1
  PWM_IN/1 -> Data Type Conversion6/1
  Data Type Conversion7/1 -> PWM_OUT/1

== system FLIGHT_Hexacopter_V2/Logging/Normalize_pwm6 ==
  In1 : Inport
  Constant : Constant  Value=1000  OutDataTypeStr=single  SampleTime=SampleTime_SAS
  Gain : Gain  Gain=1/1000
  Saturation : Saturate  UpperLimit=2000  LowerLimit=1000
  Subtract : Sum  Inputs=+-
  Out1 : Outport
  wires:
  In1/1 -> Saturation/1
  Saturation/1 -> Subtract/1
  Constant/1 -> Subtract/2
  Subtract/1 -> Gain/1
  Gain/1 -> Out1/1

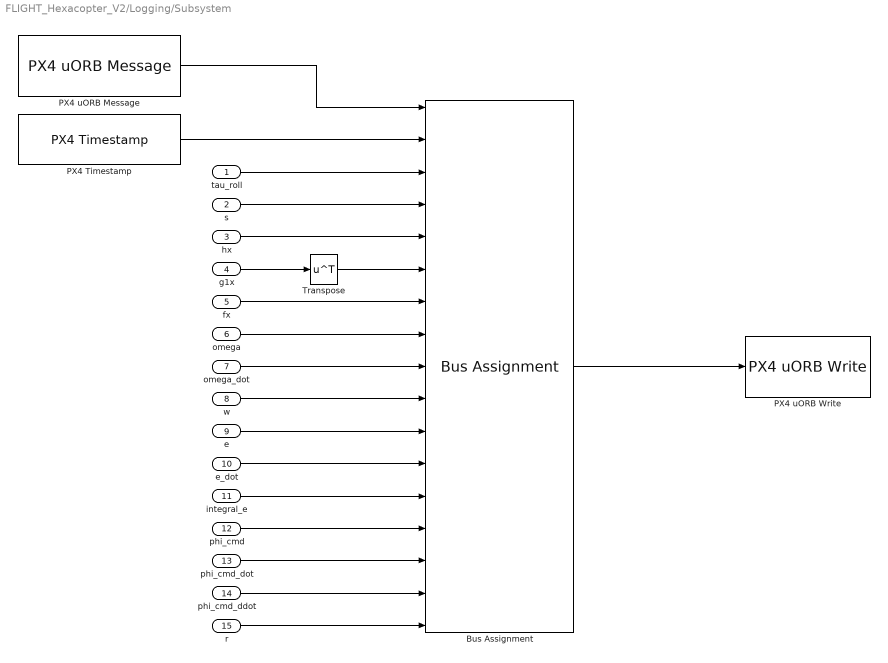
== system FLIGHT_Hexacopter_V2/Logging/Subsystem ==
  tau_roll : Inport
  s : Inport  Port=2
  hx : Inport  Port=3
  g1x : Inport  Port=4
  fx : Inport  Port=5
  omega : Inport  Port=6  PortDimensions=[1 3]
  omega_dot : Inport  Port=7
  w : Inport  Port=8
  e : Inport  Port=9
  e_dot : Inport  Port=10
  integral_e : Inport  Port=11
  phi_cmd : Inport  Port=12
  phi_cmd_dot : Inport  Port=13
  phi_cmd_ddot : Inport  Port=14
  r : Inport  Port=15
  Bus Assignment : BusAssignment  AssignedSignals=timestamp,tau_roll,s,hx,g1x,fx,omega,omega_dot,w,e,e_dot,integral_e,phi_cmd,phi_cmd_dot,phi_cmd_ddot,r
  PX4 Timestamp : px4Utilslib/PX4 Timestamp  SampleTime=SampleTime_SAS
  PX4 uORB Message : px4uORBlib/PX4 uORB Message  uORBTopic=VehicleAttitudeSmcSetpoint  SampleTime=SampleTime_SAS  selectInstance=VehicleAttitudeSmcSetpoint
  PX4 uORB Write : px4uORBlib/PX4 uORB Write  uORBTopic=VehicleAttitudeSmcSetpoint  selectInstance=VehicleAttitudeSmcSetpoint  MessageQueueLen=1
  Transpose : Math  Operator=transpose
  wires:
  Bus Assignment/1 -> PX4 uORB Write/1
  phi_cmd_dot/1 -> Bus Assignment/15
  phi_cmd/1 -> Bus Assignment/14
  integral_e/1 -> Bus Assignment/13
  PX4 uORB Message/1 -> Bus Assignment/1
  PX4 Timestamp/1 -> Bus Assignment/2
  s/1 -> Bus Assignment/4
  hx/1 -> Bus Assignment/5
  omega_dot/1 -> Bus Assignment/9
  phi_cmd_ddot/1 -> Bus Assignment/16
  g1x/1 -> Transpose/1
  r/1 -> Bus Assignment/17
  tau_roll/1 -> Bus Assignment/3
  omega/1 -> Bus Assignment/8
  e/1 -> Bus Assignment/11
  fx/1 -> Bus Assignment/7
  w/1 -> Bus Assignment/10
  e_dot/1 -> Bus Assignment/12
  Transpose/1 -> Bus Assignment/6

== system FLIGHT_Hexacopter_V2/OFP/NED2Body1 ==
  NED : Inport
  Heading : Inport  Port=2
  Calculate Transformation Matrix : Subsystem
  MatrixMultiply : Product  Multiplication=Matrix(*)
  BODY : Outport
  wires:
  Calculate Transformation Matrix/1(R) -> MatrixMultiply/1
  Heading/1 -> Calculate Transformation Matrix/1(theta)
  NED/1 -> MatrixMultiply/2
  MatrixMultiply/1 -> BODY/1

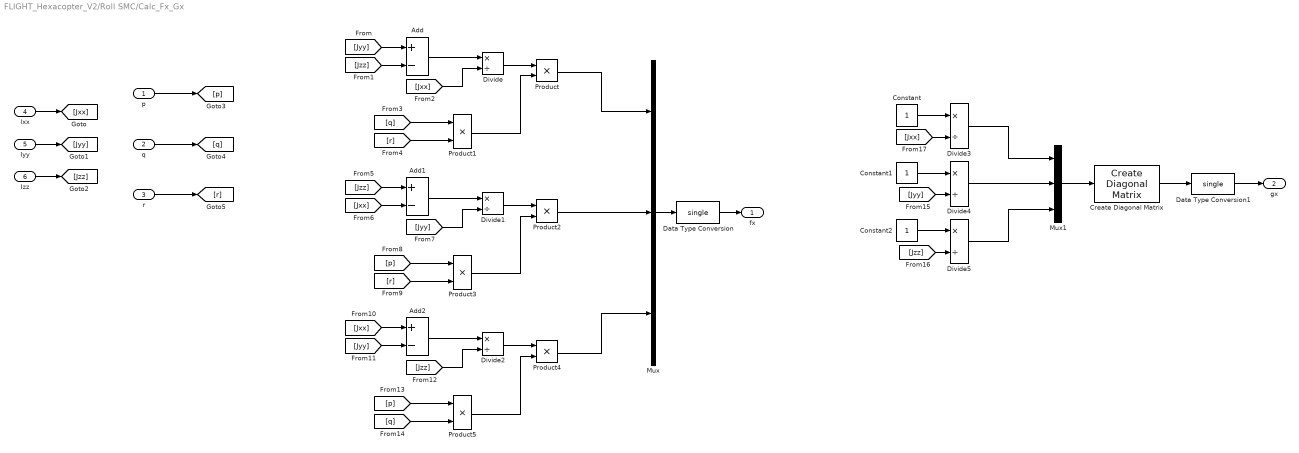
== system FLIGHT_Hexacopter_V2/Roll SMC/Calc_Fx_Gx ==
  p : Inport
  q : Inport  Port=2
  r : Inport  Port=3
  Ixx : Inport  Port=4
  Iyy : Inport  Port=5
  Izz : Inport  Port=6
  Add : Sum  Inputs=+-
  Add1 : Sum  Inputs=+-
  Add2 : Sum  Inputs=+-
  Constant : Constant  SampleTime=SampleTime_SAS
  Constant1 : Constant  SampleTime=SampleTime_SAS
  Constant2 : Constant  SampleTime=SampleTime_SAS
  Create Diagonal Matrix : matrix_library/Create Diagonal Matrix
  Data Type Conversion : DataTypeConversion  OutDataTypeStr=single  SaturateOnIntegerOverflow=off  RndMeth=Floor
  Data Type Conversion1 : DataTypeConversion  OutDataTypeStr=single  SaturateOnIntegerOverflow=off  RndMeth=Floor
  Divide{,1..5} (6 alike) : Product  Inputs=*/
  Mux : Mux  Inputs=3
  Mux1 : Mux  Inputs=3
  Product{,1..5} (6 alike) : Product
  fx : Outport
  gx : Outport  Port=2
  wires:
  Ixx/1 -> [Jxx]
  Iyy/1 -> [Jyy]
  Izz/1 -> [Jzz]
  [Jyy] -> Add/1
  [Jzz] -> Add/2
  Add/1 -> Divide/1
  [Jxx] -> Divide/2
  Divide/1 -> Product/1
  p/1 -> [p]
  q/1 -> [q]
  r/1 -> [r]
  [q] -> Product1/1
  [r] -> Product1/2
  Product1/1 -> Product/2
  Product/1 -> Mux/1
  [p] -> Product3/1
  Product2/1 -> Mux/2
  [r] -> Product3/2
  [Jzz] -> Add1/1
  Add1/1 -> Divide1/1
  Product3/1 -> Product2/2
  [Jxx] -> Add1/2
  Divide1/1 -> Product2/1
  [Jyy] -> Divide1/2
  [Jyy] -> Add2/2
  Divide2/1 -> Product4/1
  [Jxx] -> Add2/1
  Product5/1 -> Product4/2
  [q] -> Product5/2
  [p] -> Product5/1
  Add2/1 -> Divide2/1
  Product4/1 -> Mux/3
  [Jzz] -> Divide2/2
  Mux/1 -> Data Type Conversion/1
  Create Diagonal Matrix/1 -> Data Type Conversion1/1
  Mux1/1 -> Create Diagonal Matrix/1
  Data Type Conversion/1 -> fx/1
  Data Type Conversion1/1 -> gx/1
  [Jxx] -> Divide3/2
  Constant/1 -> Divide3/1
  [Jyy] -> Divide4/2
  [Jzz] -> Divide5/2
  Constant2/1 -> Divide5/1
  Constant1/1 -> Divide4/1
  Divide3/1 -> Mux1/1
  Divide4/1 -> Mux1/2
  Divide5/1 -> Mux1/3

== system FLIGHT_Hexacopter_V2/ControlAllocation(CA)/Fault_Injection/Send Fault Injection to QGC ==
  Inject : Inport
  Bus Assignment : BusAssignment  AssignedSignals=timestamp,id,event_sequence,arguments,log_levels
  PX4 Timestamp : px4Utilslib/PX4 Timestamp  SampleTime=SampleTime
  PX4 uORB Message : px4uORBlib/PX4 uORB Message  uORBTopic=Event  SampleTime=inf  selectInstance=Event
  PX4 uORB Write : px4uORBlib/PX4 uORB Write  uORBTopic=FailsafeFlags  selectInstance=FailsafeFlags  MessageQueueLen=1
  wires:
  PX4 uORB Message/1 -> Bus Assignment/1
  Bus Assignment/1 -> PX4 uORB Write/1
  PX4 Timestamp/1 -> Bus Assignment/2

== system FLIGHT_Hexacopter_V2/OFP/NED2Body1/Calculate Transformation Matrix ==
  theta : Inport
  Gain : Gain  Gain=-1
  Matrix Concatenate : Concatenate  Mode=Multidimensional array
  Mux : Mux  Inputs=2
  Mux1 : Mux  Inputs=2
  Reshape : Reshape  OutputDimensionality=Row vector (2-D)
  Reshape1 : Reshape  OutputDimensionality=Row vector (2-D)
  SinCos : Trigonometry  Operator=sincos
  Transpose : Math  Operator=transpose
  R : Outport
  wires:
  Reshape1/1 -> Matrix Concatenate/2
  Reshape/1 -> Matrix Concatenate/1
  Transpose/1 -> R/1
  Matrix Concatenate/1 -> Transpose/1
  Mux1/1 -> Reshape1/1
  Mux/1 -> Reshape/1
  Gain/1 -> Mux/2
  SinCos/1 -> Mux1/1, Gain/1
  SinCos/2 -> Mux/1, Mux1/2
  theta/1 -> SinCos/1

== matlab function FLIGHT_Hexacopter_V2/OFP/genDesireX1 ==
  data: des_v input uint64; des_x output single; v input single; x input single; reset input
function des_x = fcn(des_v, v, x, reset)
persistent prev_reset;

if(abs(des_v) < 0.001) % integrator reset condition
    if(abs(v) <= 2) % 1 m/s 이내라면 즉시 정지
        des_x = x;

    else(abs(v) > 2) % 1m/s 이상이라면
        des_x = x + v;
    end
        
else
    des_x = x; % feedforward Only
end

== matlab function FLIGHT_Hexacopter_V2/OFP/MATLAB Function3 ==
  data: vy_b input; vx_b input; vx_i output; heading input; vy_i output
function [vx_i, vy_i] = axisTransform(vy_b, vx_b, heading)

R_b2i = [cos(heading), -sin(heading); sin(heading), cos(heading)]; %body to inertia

V = R_b2i * [vx_b; vy_b];

vx_i = V(1);
vy_i = V(2);

== matlab function FLIGHT_Hexacopter_V2/OFP/MATLAB Function4 ==
  data: des_theta output; a_cmd input; des_phi output; heading input
function [des_theta, des_phi] = acc2attitude(a_cmd, heading)
g = 9.81; 
d2r = pi/180;

R_psi_inv= [sin(heading), -cos(heading); cos(heading), sin(heading)];

Theta = -1/g * R_psi_inv * a_cmd;

des_phi = min(Theta(1), 20*d2r);
des_theta = min(Theta(2), 20*d2r);

== matlab function FLIGHT_Hexacopter_V2/OFP/WPManager ==
  data: X input; Current_WP output; heading input; L input; flag input
function Current_WP = WPManager(X, heading, L, flag)

% X: Current Position NED
% L: Length of Square Waypoint
% flag: Engage WP Flight

persistent X0
if(isempty(X0))
    X0 = [0,0];
end
persistent WP_num
if(isempty(WP_num))
    WP_num=0;
end
persistent WP
if(isempty(WP))
    WP = [0 0; 0 0; 0 0; 0 0; 0 0]';
end


%%%%%% Code %%%%%%%

if(flag) % Engage WP Flight
    % Generate WP first Time
    if(WP_num < 1)

        R_b2i = [cos(heading), -sin(heading); sin(heading), cos(heading)]; %body to inertia

        WP_b = [
        X0(1),X0(2); 
        X0(1)+L,X0(2); 
        X0(1)+L,X0(2)+L; 
        X0(1), X0(2)+L;
        X0(1), X0(2)];
        WP = R_b2i * WP_b';
    end
    WP_idx = rem(WP_num, length(WP)) + 1;
    Current_WP = WP(:,WP_idx);
    distance = sqrt((Current_WP(1)-X(1))^2 + (Current_WP(2)-X(2))^2);

    if(distance < 0.5) % 0.2m 이내라면
        WP_num = WP_num+1;
    end
    

else % Stop
    X0 = [0, 0]; % Update Reference Position
    WP_num = 0; % Reset WP Order
    Current_WP = X0';

end

== matlab function FLIGHT_Hexacopter_V2/Roll SMC/MATLAB Function1 ==
  data: omega input; G1 output; gx input; kd input
function G1 = G(omega, gx, kd)

G1 = kd*omega * gx;

== matlab function FLIGHT_Hexacopter_V2/Roll SMC/MATLAB Function2 ==
  data: Hx input; u output; G1x input; R input; G1_inv output
function [u,G1_inv] = U(Hx, G1x, R)

G1_inv = pinv(G1x);

u = G1_inv * (-Hx + R);

== matlab function FLIGHT_Hexacopter_V2/Roll SMC/MATLAB Function3 ==
  data: e input; s output; e_dot input; integral_e input; kp input; ki input; kd input
function s = SlidingSurface(e, e_dot, integral_e, kp, ki, kd)

% PID Like Sliding Surface

s = kd*e_dot + kp*e + ki*integral_e;

== matlab function FLIGHT_Hexacopter_V2/Roll SMC/MATLAB Function4 ==
  data: ST_R output; s input; R output; ks input; kp input; eps input; lamda input; eta input; w input single; wdot output
function [ST_R,R,wdot] = ReachingLaw(s, ks, kp, eps, lamda, eta, w)

% Sign Function
%R = -ks*sign(s) - kp*s;

% Modified Sigmoid
R = -ks*( s/(abs(s)+eps) ) - kp*s;

% Super-Twisting 
u1 = -lamda*abs(s)^0.5*sign(s)-w;
wdot = single(eta*sign(s));
ST_R = u1;

== matlab function FLIGHT_Hexacopter_V2/Parameters_PARAMS/MATLAB Function ==
  data: w_hz input; w_radps output
function w_radps= hz2radps(w_hz)

w_radps = w_hz * 2*pi;

== matlab function FLIGHT_Hexacopter_V2/Roll SMC/Omega_phi ==
  data: phi input; omega_phi output; theta input
function omega_phi  = CalcOmega(phi, theta)

omega_phi = [1, sin(phi)*tan(theta), cos(phi)*tan(theta)];

== matlab function FLIGHT_Hexacopter_V2/OFP/MATLAB Function1 ==
  data: in_roll input double; in_pitch input double; in_yawrate input double; flag input boolean; out_roll output double; out_pitch output double; out_yawrate output double; time_usec input double; peak_angle_deg input double; doublet_dt input double; doublet_axis input int32
function [out_roll, out_pitch,out_yawrate]= DoubletGenerator(in_roll, in_pitch, in_yawrate, flag, time_usec, peak_angle_deg, doublet_dt, doublet_axis)
persistent start_time_usec;
if(isempty(start_time_usec))
    start_time_usec = -1;
end

if(flag && start_time_usec == -1)
    start_time_usec = time_usec;
end
d2r = pi/180;

if (flag && start_time_usec > 0) % time calculation
    reletive_time_sec = double(time_usec - start_time_usec)*1e-6;
else
    start_time_usec = -1;
    reletive_time_sec = 0;
end

% Define Doublet
t1 = 0;
t2 = t1+doublet_dt;
t3 = t2+doublet_dt;
peak_angle_rad = peak_angle_deg * d2r;

% Default Output
out_roll = in_roll;
out_pitch = in_pitch;
out_yawrate = in_yawrate;

% Generate Doublet Command
if(flag)
    if(reletive_time_sec >= t1 && reletive_time_sec < t2)
        cmd = peak_angle_rad;
    elseif(reletive_time_sec >= t2 && reletive_time_sec < t3)
        cmd = -peak_angle_rad;
    else
        cmd = 0;
    end

    switch(double(doublet_axis))
        case 1
            out_roll = cmd;
        case 2
            out_pitch = cmd;
        case 3
            out_yawrate = cmd;
    end
end

== matlab function FLIGHT_Hexacopter_V2/OFP/MATLAB Function ==
  data: stab_u input; y output; alt_u input; pos_u input; mode input; flag_pos_mode input; flag_alt_mode input
function y = flightmode(stab_u, alt_u, pos_u, mode, flag_pos_mode, flag_alt_mode)

if(mode >= 1800 && flag_pos_mode) % position
    y = pos_u;
elseif(mode <1800 && mode >=1400 && flag_alt_mode) % Altitude
    y = alt_u;
else % Stablized
    y = stab_u;
end

== matlab function FLIGHT_Hexacopter_V2/Read_uORB(250hz)_SENSORS250/quat2eul ==
  data: q input; ypr output
function ypr  = quat2eul(q)

% Quaternion conversion to Euler angles based on the PX4 Firmware v1.10.2
% release.

phi = atan2(2*(q(1)*q(2) + q(3)* q(4)), q(1)^2 - q(2)^2 - q(3)^2 + q(4)^2);
theta = asin(-2*(q(2)*q(4) - q(1)*q(3)));
psi = atan2(2*(q(2)*q(3) + q(1)* q(4)), q(1)^2 + q(2)^2 - q(3)^2 - q(4)^2);

ypr = [psi theta phi];

end

== matlab function FLIGHT_Hexacopter_V2/Read_uORB(250hz)_SENSORS250/MATLAB Function ==
  data: nav_stat input; flag_stab output; flag_alt output; flag_pos output
function [flag_stab, flag_alt, flag_pos] = flightmode(nav_stat)

if(nav_stat == 1) % ALT Mode
    flag_pos = false;
    flag_alt = true;
    flag_stab = false;

elseif(nav_stat == 2) % POS Mode
    flag_pos = true;
    flag_alt = false;
    flag_stab = false;

else % STAB mode
    flag_pos = false;
    flag_alt = false;
    flag_stab = true;
end

== matlab function FLIGHT_Hexacopter_V2/OFP/MATLAB Function2 ==
  data: a_z input; des_throttle output; thr_hover input
function des_throttle = fcn(a_z, thr_hover)

des_throttle = thr_hover - a_z/9.81;

== matlab function FLIGHT_Hexacopter_V2/Roll SMC/MATLAB Function ==
  data: omega_dot input; omega input; H output; w input; fx input; phi_cmd_ddot input; phi_cmd_dot input; e input; kp input; ki input; kd input
function H = H(omega_dot, omega, w, fx, phi_cmd_ddot, phi_cmd_dot, e, kp,ki,kd)

phi_cmd_ddot = 0; % Suppose
H = kd*(omega_dot*w + omega*fx - phi_cmd_ddot) + kp*(omega*w - phi_cmd_dot) + ki*e;

== matlab function FLIGHT_Hexacopter_V2/OFP/genDesireX ==
  data: des_v input single; des_x output single; v input single; x input single; reset input boolean; timestamp input uint64
function des_x = fcn(des_v, v, x, reset, timestamp)
persistent prev_time
persistent prev_reset;


if(isempty(prev_time))
    prev_time = timestamp;
end
if(isempty(prev_reset))
    prev_reset = reset;
end


dt = double(timestamp-prev_time)*1e-6; % us to sec

if(prev_reset ~= reset) % integrator reset condition
    if(abs(v) <= 2) % 1 m/s 이내라면 즉시 정지
        des_x = x;
        prev_reset = reset;

    else(abs(v) > 2) % 1m/s 이상이라면
        des_x = x + v;
        prev_reset = reset;
    end
    prev_time = timestamp;
        
else
    des_x = x + des_v*dt;
    des_x = cast(des_x,'single');
    prev_time = timestamp;
end
